simulink model "xy_frequency"  (R2018a)
settings: Solver=VariableStepAuto  StartTime=0.0  StopTime=20  RelTol=1e-3
undefined symbols (not defined in the file): drone, est_c_A, est_c_B, est_c_C, est_c_D, matrix_xA, matrix_xB, matrix_xC, matrix_xD, matrix_yA, matrix_yB, matrix_yC, matrix_yD, regulator_gain_of_attitude, simulation_sampling_ts, vd, vi, vp, xp, yp
libraries: simulink x3
settings Model: Creator=ros  LastModifiedBy=ros

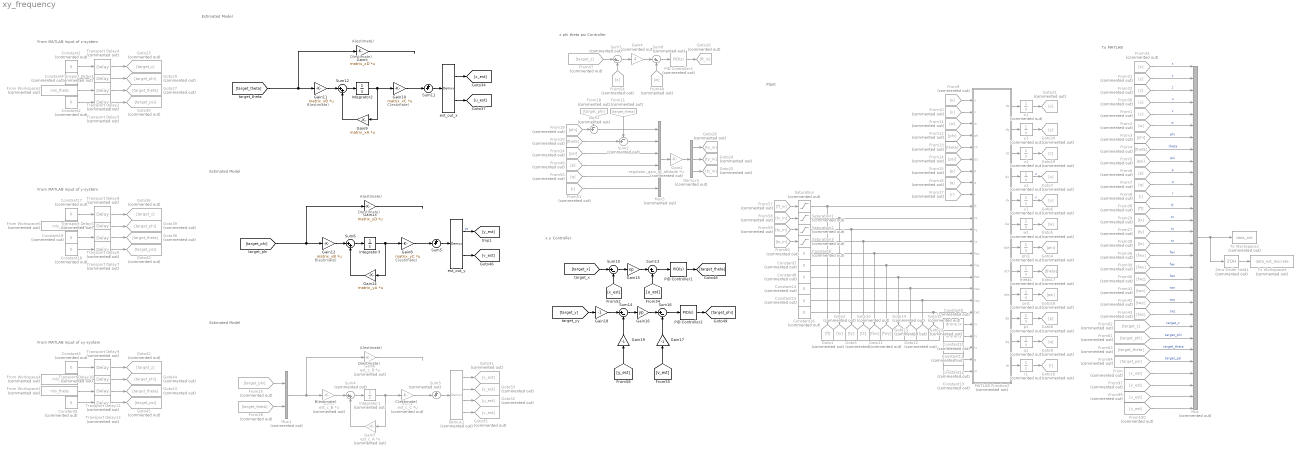
== system xy_frequency ==
  note: To MATLAB
  note: Estimated Model
  note: A(estimate)
  note: B(estimate)
  note: C(estimate)
  note: D(estimate)
  note: z phi theta psi Controller
  note: Plant
  note: D(estimate)
  note: A(estimate)
  note: B(estimate)
  note: Estimated Model
  note: C(estimate)
  note: From MATLAB Input of xy-system
  note: From MATLAB Input of x-system
  note: A(estimate)
  note: B(estimate)
  note: Estimated Model
  note: D(estimate)
  note: C(estimate)
  note: From MATLAB Input of y-system
  note: x y Controller
  Constant{1..8,14..19} (14 alike) : Constant  Commented=on  Value=0
  Constant10 : Constant  Commented=on  Value=drone.Iy
  Constant11 : Constant  Commented=on  Value=drone.Iz
  Constant12 : Constant  Commented=on  Value=drone.g
  Constant13 : Constant  Commented=on  Value=drone.m
  Constant9 : Constant  Commented=on  Value=drone.Ix
  Demux1 : Demux  Commented=on
  Demux5 : Demux  Commented=on  Outputs=3
  From : From  Commented=on  GotoTag=x_est
  From Workspace1 : FromWorkspace  Commented=on  VariableName=mls_theta  SampleTime=0
  From Workspace2 : FromWorkspace  Commented=on  VariableName=mls_theta  SampleTime=0
  From Workspace4 : FromWorkspace  Commented=on  VariableName=mls_phi  SampleTime=0
  From Workspace5 : FromWorkspace  Commented=on  VariableName=mls_phi  SampleTime=0
  From1 : From  Commented=on  GotoTag=v
  From10 : From  Commented=on  GotoTag=v
  From100 : From  Commented=on  GotoTag=v_est
  From11 : From  Commented=on  GotoTag=w
  From12 : From  Commented=on  GotoTag=phi
  From13 : From  Commented=on  GotoTag=theta
  From14 : From  Commented=on  GotoTag=psi
  From15 : From  Commented=on  GotoTag=p
  From16 : From  Commented=on  GotoTag=q
  From17 : From  Commented=on  GotoTag=r
  From18 : From  Commented=on  GotoTag=target_phi
  From19 : From  Commented=on  GotoTag=phi
  From2 : From  Commented=on  GotoTag=w
  From20 : From  Commented=on  GotoTag=theta
  From21 : From  Commented=on  GotoTag=target_theta
  From24 : From  Commented=on  GotoTag=psi
  From25 : From  Commented=on  GotoTag=target_phi
  From26 : From  Commented=on  GotoTag=target_theta
  From27 : From  Commented=on  GotoTag=ty
  From28 : From  Commented=on  GotoTag=tz
  From29 : From  Commented=on  GotoTag=tx
  From3 : From  Commented=on  GotoTag=phi
  From30 : From  Commented=on  GotoTag=u
  From31 : From  Commented=on  GotoTag=y
  From32 : From  Commented=on  GotoTag=z
  From33 : From  Commented=on  GotoTag=x
  From36 : From  Commented=on  GotoTag=fwx
  From38 : From  Commented=on  GotoTag=ft
  From39 : From  Commented=on  GotoTag=fwy
  From4 : From  Commented=on  GotoTag=theta
  From40 : From  Commented=on  GotoTag=fwz
  From41 : From  Commented=on  GotoTag=twx
  From42 : From  Commented=on  GotoTag=twy
  From43 : From  Commented=on  GotoTag=twz
  From47 : From  Commented=on  GotoTag=target_z
  From48 : From  Commented=on  GotoTag=w
  From49 : From  Commented=on  GotoTag=p
  From5 : From  Commented=on  GotoTag=psi
  From50 : From  Commented=on  GotoTag=q
  From51 : From  Commented=on  GotoTag=r
  From54 : From  Commented=on  GotoTag=z
  From57 : From  Commented=on  GotoTag=ft_in
  From58 : From  Commented=on  GotoTag=tx_in
  From59 : From  Commented=on  GotoTag=ty_in
  From6 : From  Commented=on  GotoTag=p
  From60 : From  Commented=on  GotoTag=tz_in
  From61 : From  Commented=on  GotoTag=target_phi
  From62 : From  Commented=on  GotoTag=target_z
  From63 : From  Commented=on  GotoTag=target_theta
  From64 : From  Commented=on  GotoTag=target_psi
  From7 : From  Commented=on  GotoTag=q
  From8 : From  Commented=on  GotoTag=r
  From9 : From  Commented=on  GotoTag=u
  From97 : From  Commented=on  GotoTag=y_est
  From99 : From  Commented=on  GotoTag=u_est
  Gain1 : Gain  Commented=on  Gain=-regulator_gain_of_attitude  Multiplication=Matrix(K*u)
  Gain10 : Gain  Gain=matrix_xC  Multiplication=Matrix(K*u)
  Gain11 : Gain  Gain=matrix_xB  Multiplication=Matrix(K*u)
  Gain12 : Gain  Gain=matrix_yB  Multiplication=Matrix(K*u)
  Gain13 : Gain  Gain=matrix_yD  Multiplication=Matrix(K*u)
  Gain14 : Gain  Gain=matrix_yA  Multiplication=Matrix(K*u)
  Gain15 : Gain  Gain=xp
  Gain16 : Gain  Gain=yp
  Gain17 : Gain  Gain=-1
  Gain18 : Gain  Gain=-1
  Gain19 : Gain  Gain=-1
  Gain2 : Gain  Commented=on  Gain=est_c_C  Multiplication=Matrix(K*u)
  Gain3 : Gain  Commented=on  Gain=est_c_B  Multiplication=Matrix(K*u)
  Gain4 : Gain  Commented=on  Gain=4
  Gain5 : Gain  Gain=matrix_xD  Multiplication=Matrix(K*u)
  Gain6 : Gain  Commented=on  Gain=est_c_D  Multiplication=Matrix(K*u)
  Gain7 : Gain  Commented=on  Gain=est_c_A  Multiplication=Matrix(K*u)
  Gain8 : Gain  Gain=matrix_yC  Multiplication=Matrix(K*u)
  Gain9 : Gain  Gain=matrix_xA  Multiplication=Matrix(K*u)
  Goto1 : Goto  Commented=on  GotoTag=ft
  Goto10 : Goto  Commented=on  GotoTag=tz
  Goto11 : Goto  Commented=on  GotoTag=fwx
  Goto12 : Goto  Commented=on  GotoTag=twx
  Goto13 : Goto  Commented=on  GotoTag=fwy
  Goto14 : Goto  Commented=on  GotoTag=fwz
  Goto15 : Goto  Commented=on  GotoTag=twz
  Goto16 : Goto  Commented=on  GotoTag=r
  Goto17 : Goto  Commented=on  GotoTag=theta
  Goto18 : Goto  Commented=on  GotoTag=psi
  Goto19 : Goto  Commented=on  GotoTag=z
  Goto2 : Goto  Commented=on  GotoTag=tx
  Goto20 : Goto  Commented=on  GotoTag=y
  Goto21 : Goto  Commented=on  GotoTag=x
  Goto22 : Goto  Commented=on  GotoTag=twy
  Goto23 : Goto  Commented=on  GotoTag=target_z
  Goto24 : Goto  Commented=on  GotoTag=ty_in
  Goto25 : Goto  Commented=on  GotoTag=tz_in
  Goto26 : Goto  Commented=on  GotoTag=ft_in
  Goto27 : Goto  Commented=on  GotoTag=target_theta
  Goto28 : Goto  Commented=on  GotoTag=tx_in
  Goto29 : Goto  Commented=on  GotoTag=target_phi
  Goto3 : Goto  Commented=on  GotoTag=ty
  Goto30 : Goto  Commented=on  GotoTag=target_psi
  Goto31 : Goto  Commented=on  GotoTag=x_est
  Goto32 : Goto  Commented=on  GotoTag=u_est
  Goto33 : Goto  Commented=on  GotoTag=y_est
  Goto35 : Goto  Commented=on  GotoTag=v_est
  Goto36 : Goto  Commented=on  GotoTag=target_z
  Goto38 : Goto  Commented=on  GotoTag=target_theta
  Goto39 : Goto  Commented=on  GotoTag=target_phi
  Goto4 : Goto  Commented=on  GotoTag=phi
  Goto40 : Goto  Commented=on  GotoTag=target_psi
  Goto42 : Goto  Commented=on  GotoTag=target_z
  Goto43 : Goto  Commented=on  GotoTag=target_theta
  Goto44 : Goto  Commented=on  GotoTag=target_phi
  Goto45 : Goto  Commented=on  GotoTag=target_psi
  Goto5 : Goto  Commented=on  GotoTag=w
  Goto6 : Goto  Commented=on  GotoTag=v
  Goto7 : Goto  Commented=on  GotoTag=u
  Goto8 : Goto  Commented=on  GotoTag=p
  Goto9 : Goto  Commented=on  GotoTag=q
  Integrator1 : Integrator  Commented=on
  Integrator2 : Integrator
  Integrator3 : Integrator
  MATLAB Function2 : MATLAB Function  Commented=on  TreatAsAtomicUnit=on
  Mux : Mux  Commented=on  Inputs=30
  Mux1 : Mux  Commented=on  Inputs=2
  Mux5 : Mux  Commented=on  Inputs=6
  PID Controller1 : simulink/Continuous/PID Controller  Controller=PID  TimeDomain=Continuous-time  SampleTime=-1  IntegratorMethod=Forward Euler  FilterMethod=Forward Euler  Form=Parallel  UseFilter=on  ControllerParametersSource=internal  P=vp  I=vi  D=vd  N=100  InitialConditionSource=internal  InitialConditionForIntegrator=0  InitialConditionForFilter=0  ExternalReset=none  LimitOutput=off  UpperSaturationLimit=inf  LowerSaturationLimit=-inf  LinearizeAsGain=on  AntiWindupMode=none  Kb=1  TrackingMode=off  Kt=1  PParamMin=[]  PParamMax=[]  IParamMin=[]  IParamMax=[]  DParamMin=[]  DParamMax=[]  NParamMin=[]  NParamMax=[]  KbParamMin=[]  KbParamMax=[]  KtParamMin=[]  KtParamMax=[]  POutMin=[]  POutMax=[]  IOutMin=[]  IOutMax=[]  DOutMin=[]  DOutMax=[]  NOutMin=[]  NOutMax=[]  KbOutMin=[]  KbOutMax=[]  KtOutMin=[]  KtOutMax=[]  IntegratorOutMin=[]  IntegratorOutMax=[]  FilterOutMin=[]  FilterOutMax=[]  SumOutMin=[]  SumOutMax=[]  SumI1OutMin=[]  SumI1OutMax=[]  SumI2OutMin=[]  SumI2OutMax=[]  SumI3OutMin=[]  SumI3OutMax=[]  SumDOutMin=[]  SumDOutMax=[]  SaturationOutMin=[]  SaturationOutMax=[]  IntegratorContinuousStateAttributes=''  IntegratorStateMustResolveToSignalObject=off  IntegratorRTWStateStorageClass=Auto  FilterContinuousStateAttributes=''  FilterStateMustResolveToSignalObject=off  FilterRTWStateStorageClass=Auto  DifferentiatorICPrevScaledInput=0  DifferentiatorOutMin=[]  DifferentiatorOutMax=[]  FilterDiffOutCoefMin=[]  FilterDiffOutCoefMax=[]  SumDenOutMin=[]  SumDenOutMax=[]  SumNumOutMin=[]  SumNumOutMax=[]  ReciprocalOutMin=[]  ReciprocalOutMax=[]  DivideOutMin=[]  DivideOutMax=[]  TunerSelectOption=Transfer Function Based (PID Tuner App)
  PID Controller2 : simulink/Continuous/PID Controller  Controller=PID  TimeDomain=Continuous-time  SampleTime=-1  IntegratorMethod=Forward Euler  FilterMethod=Forward Euler  Form=Parallel  UseFilter=on  ControllerParametersSource=internal  P=vp  I=vi  D=vd  N=113.724914636651  InitialConditionSource=internal  InitialConditionForIntegrator=0  InitialConditionForFilter=0  ExternalReset=none  LimitOutput=off  UpperSaturationLimit=inf  LowerSaturationLimit=-inf  LinearizeAsGain=on  AntiWindupMode=none  Kb=1  TrackingMode=off  Kt=1  PParamMin=[]  PParamMax=[]  IParamMin=[]  IParamMax=[]  DParamMin=[]  DParamMax=[]  NParamMin=[]  NParamMax=[]  KbParamMin=[]  KbParamMax=[]  KtParamMin=[]  KtParamMax=[]  POutMin=[]  POutMax=[]  IOutMin=[]  IOutMax=[]  DOutMin=[]  DOutMax=[]  NOutMin=[]  NOutMax=[]  KbOutMin=[]  KbOutMax=[]  KtOutMin=[]  KtOutMax=[]  IntegratorOutMin=[]  IntegratorOutMax=[]  FilterOutMin=[]  FilterOutMax=[]  SumOutMin=[]  SumOutMax=[]  SumI1OutMin=[]  SumI1OutMax=[]  SumI2OutMin=[]  SumI2OutMax=[]  SumI3OutMin=[]  SumI3OutMax=[]  SumDOutMin=[]  SumDOutMax=[]  SaturationOutMin=[]  SaturationOutMax=[]  IntegratorContinuousStateAttributes=''  IntegratorStateMustResolveToSignalObject=off  IntegratorRTWStateStorageClass=Auto  FilterContinuousStateAttributes=''  FilterStateMustResolveToSignalObject=off  FilterRTWStateStorageClass=Auto  DifferentiatorICPrevScaledInput=0  DifferentiatorOutMin=[]  DifferentiatorOutMax=[]  FilterDiffOutCoefMin=[]  FilterDiffOutCoefMax=[]  SumDenOutMin=[]  SumDenOutMax=[]  SumNumOutMin=[]  SumNumOutMax=[]  ReciprocalOutMin=[]  ReciprocalOutMax=[]  DivideOutMin=[]  DivideOutMax=[]  TunerSelectOption=Transfer Function Based (PID Tuner App)
  PID Controller3 : simulink/Continuous/PID Controller  Commented=on  Controller=PID  TimeDomain=Continuous-time  SampleTime=-1  IntegratorMethod=Forward Euler  FilterMethod=Forward Euler  Form=Parallel  UseFilter=on  ControllerParametersSource=internal  P=7  I=6  D=0.7  N=100  InitialConditionSource=internal  InitialConditionForIntegrator=0  InitialConditionForFilter=0  ExternalReset=none  LimitOutput=off  UpperSaturationLimit=inf  LowerSaturationLimit=-inf  LinearizeAsGain=on  AntiWindupMode=none  Kb=1  TrackingMode=off  Kt=1  PParamMin=[]  PParamMax=[]  IParamMin=[]  IParamMax=[]  DParamMin=[]  DParamMax=[]  NParamMin=[]  NParamMax=[]  KbParamMin=[]  KbParamMax=[]  KtParamMin=[]  KtParamMax=[]  POutMin=[]  POutMax=[]  IOutMin=[]  IOutMax=[]  DOutMin=[]  DOutMax=[]  NOutMin=[]  NOutMax=[]  KbOutMin=[]  KbOutMax=[]  KtOutMin=[]  KtOutMax=[]  IntegratorOutMin=[]  IntegratorOutMax=[]  FilterOutMin=[]  FilterOutMax=[]  SumOutMin=[]  SumOutMax=[]  SumI1OutMin=[]  SumI1OutMax=[]  SumI2OutMin=[]  SumI2OutMax=[]  SumI3OutMin=[]  SumI3OutMax=[]  SumDOutMin=[]  SumDOutMax=[]  SaturationOutMin=[]  SaturationOutMax=[]  IntegratorContinuousStateAttributes=''  IntegratorStateMustResolveToSignalObject=off  IntegratorRTWStateStorageClass=Auto  FilterContinuousStateAttributes=''  FilterStateMustResolveToSignalObject=off  FilterRTWStateStorageClass=Auto  DifferentiatorICPrevScaledInput=0  DifferentiatorOutMin=[]  DifferentiatorOutMax=[]  FilterDiffOutCoefMin=[]  FilterDiffOutCoefMax=[]  SumDenOutMin=[]  SumDenOutMax=[]  SumNumOutMin=[]  SumNumOutMax=[]  ReciprocalOutMin=[]  ReciprocalOutMax=[]  DivideOutMin=[]  DivideOutMax=[]  TunerSelectOption=Transfer Function Based (PID Tuner App)
  Saturation{,1..3} (4 alike) : Saturate  Commented=on  UpperLimit=30  LowerLimit=-100
  Sum1 : Sum  Commented=on  Inputs=-+|
  Sum{10,13..14,16} (4 alike) : Sum  Inputs=|+-
  Sum11 : Sum  Inputs=++|
  Sum12 : Sum  Inputs=|++
  Sum2 : Sum  Commented=on  Inputs=-+|
  Sum3 : Sum  Commented=on  Inputs=++|
  Sum4 : Sum  Commented=on  Inputs=|++
  Sum5 : Sum  Inputs=++|
  Sum6 : Sum  Inputs=|++
  Sum7 : Sum  Commented=on  Inputs=|+-
  Sum8 : Sum  Commented=on  Inputs=|+-
  To Workspace2 : ToWorkspace  Commented=on  VariableName=data_est  SaveFormat=Timeseries  SampleTime=-1
  To Workspace4 : ToWorkspace  Commented=on  VariableName=data_est_discrete  SaveFormat=Timeseries  SampleTime=-1
  Transport Delay{1..12} (12 alike) : TransportDelay  Commented=on  DelayTime=10
  Zero-Order Hold1 : ZeroOrderHold  Commented=on  SampleTime=simulation_sampling_ts
  est_out_x : Demux  Outputs=2
  est_out_y : Demux  Tag=dfd  Outputs=2
  p1 : Integrator  Commented=on
  phi1 : Integrator  Commented=on
  psi1 : Integrator  Commented=on
  q1 : Integrator  Commented=on
  r1 : Integrator  Commented=on
  theta1 : Integrator  Commented=on
  u1 : Integrator  Commented=on
  v1 : Integrator  Commented=on
  w1 : Integrator  Commented=on
  x1 : Integrator  Commented=on
  y1 : Integrator  Commented=on
  z1 : Integrator  Commented=on
  wires:
  From33/1 -> Mux/1  "x"
  From1/1 -> Mux/5  "v"
  From32/1 -> Mux/3  "z"
  From2/1 -> Mux/6  "w"
  From6/1 -> Mux/10  "p"
  From3/1 -> Mux/7  "phi"
  From4/1 -> Mux/8  "theta"
  From8/1 -> Mux/12  "r"
  From31/1 -> Mux/2  "y"
  From5/1 -> Mux/9  "psi"
  From30/1 -> Mux/4  "u"
  From7/1 -> Mux/11  "q"
  Mux/1 -> Zero-Order Hold1/1, To Workspace2/1
  From38/1 -> Mux/13  "ft"
  From29/1 -> Mux/14  "tx"
  From27/1 -> Mux/15  "ty"
  From28/1 -> Mux/16  "tz"
  From36/1 -> Mux/17  "fwx"
  From39/1 -> Mux/18  "fwy"
  From40/1 -> Mux/19  "fwz"
  From41/1 -> Mux/20  "twx"
  From42/1 -> Mux/21  "twy"
  From43/1 -> Mux/22  "twz"
  Zero-Order Hold1/1 -> To Workspace4/1
  From62/1 -> Mux/23  "target_z"
  From61/1 -> Mux/24  "target_phi"
  From63/1 -> Mux/25  "target_theta"
  From64/1 -> Mux/26  "target_psi"
  From/1 -> Mux/27
  From97/1 -> Mux/28
  est_out_x/1 -> [x_est]
  Sum11/1 -> est_out_x/1
  Integrator2/1 -> Gain10/1, Gain9/1
  Gain5/1 -> ?
  Gain11/1 -> Sum12/1
  Gain9/1 -> Sum12/2
  Gain10/1 -> Sum11/2
  Sum12/1 -> Integrator2/1
  [target_theta] -> Gain5/1, Gain11/1
  est_out_x/2 -> [u_est]
  PID Controller3/1 -> Goto26/1
  From47/1 -> Sum7/1
  Sum1/1 -> Mux5/1
  Sum2/1 -> Mux5/2
  From20/1 -> Sum2/2
  Demux5/3 -> Goto25/1
  Sum8/1 -> PID Controller3/1
  From54/1 -> Sum7/2
  Demux5/2 -> Goto24/1
  From51/1 -> Mux5/6
  From50/1 -> Mux5/5
  Demux5/1 -> Goto28/1
  From19/1 -> Sum1/2
  From21/1 -> Sum2/1
  Gain1/1 -> Demux5/1
  Sum7/1 -> Gain4/1
  From18/1 -> Sum1/1
  From48/1 -> Sum8/2
  Mux5/1 -> Gain1/1
  From24/1 -> Mux5/3
  From49/1 -> Mux5/4
  Gain4/1 -> Sum8/1
  v1/1 -> Goto6/1  "v"
  MATLAB Function2/8(dth) -> theta1/1
  From57/1 -> Saturation/1
  MATLAB Function2/10(dp) -> p1/1
  Constant16/1 -> Goto15/1, MATLAB Function2/19(twz)
  MATLAB Function2/12(dr) -> r1/1
  MATLAB Function2/2(dy) -> y1/1
  Constant8/1 -> Goto14/1, MATLAB Function2/16(fwz)
  w1/1 -> Goto5/1
  MATLAB Function2/4(du) -> u1/1
  phi1/1 -> Goto4/1
  Constant15/1 -> Goto22/1, MATLAB Function2/18(twy)
  From16/1 -> MATLAB Function2/8(q)
  From60/1 -> Saturation3/1
  MATLAB Function2/7(dph) -> phi1/1
  Constant6/1 -> Goto11/1, MATLAB Function2/14(fwx)
  Saturation/1 -> Goto1/1, MATLAB Function2/10(ft)
  Saturation3/1 -> Goto10/1, MATLAB Function2/13(tz)
  From12/1 -> MATLAB Function2/4(ph)
  Constant13/1 -> MATLAB Function2/24(m)
  Constant9/1 -> MATLAB Function2/20(Ix)
  z1/1 -> Goto19/1
  q1/1 -> Goto9/1
  psi1/1 -> Goto18/1
  From17/1 -> MATLAB Function2/9(r)
  From13/1 -> MATLAB Function2/5(th)
  MATLAB Function2/5(dv) -> v1/1
  Constant12/1 -> MATLAB Function2/23(g)
  Saturation2/1 -> Goto3/1, MATLAB Function2/12(ty)
  r1/1 -> Goto16/1
  Constant7/1 -> Goto13/1, MATLAB Function2/15(fwy)
  MATLAB Function2/9(dps) -> psi1/1
  Constant11/1 -> MATLAB Function2/22(Iz)
  From15/1 -> MATLAB Function2/7(p)
  theta1/1 -> Goto17/1
  From14/1 -> MATLAB Function2/6(ps)
  x1/1 -> Goto21/1
  MATLAB Function2/3(dz) -> z1/1
  From59/1 -> Saturation2/1
  Constant10/1 -> MATLAB Function2/21(Iy)
  MATLAB Function2/11(dq) -> q1/1
  y1/1 -> Goto20/1
  From11/1 -> MATLAB Function2/3(w)
  From9/1 -> MATLAB Function2/1(u)
  From10/1 -> MATLAB Function2/2(v)
  MATLAB Function2/6(dw) -> w1/1
  u1/1 -> Goto7/1  "u"
  p1/1 -> Goto8/1
  Saturation1/1 -> Goto2/1, MATLAB Function2/11(tx)
  Constant14/1 -> Goto12/1, MATLAB Function2/17(twx)
  MATLAB Function2/1(dx) -> x1/1
  From58/1 -> Saturation1/1
  From100/1 -> Mux/30
  From99/1 -> Mux/29
  Integrator1/1 -> Gain2/1, Gain7/1
  Gain6/1 -> ?
  Demux1/1 -> Goto31/1
  Demux1/2 -> Goto33/1
  Demux1/3 -> Goto32/1
  From26/1 -> Mux1/2
  Mux1/1 -> Gain6/1, Gain3/1
  Demux1/4 -> Goto35/1
  From25/1 -> Mux1/1
  Gain2/1 -> Sum3/2
  Sum3/1 -> Demux1/1
  Sum4/1 -> Integrator1/1
  Gain3/1 -> Sum4/1
  Gain7/1 -> Sum4/2
  Constant5/1 -> Transport Delay12/1
  Constant1/1 -> Transport Delay4/1
  From Workspace1/1 -> Transport Delay11/1
  Transport Delay2/1 -> Goto27/1
  Transport Delay4/1 -> Goto23/1
  From Workspace2/1 -> Transport Delay2/1
  Transport Delay10/1 -> Goto44/1
  Transport Delay3/1 -> Goto30/1
  Constant4/1 -> Transport Delay1/1
  Transport Delay11/1 -> Goto43/1
  Transport Delay1/1 -> Goto29/1
  Transport Delay9/1 -> Goto42/1
  Constant3/1 -> Transport Delay9/1
  Constant2/1 -> Transport Delay3/1
  From Workspace4/1 -> Transport Delay10/1
  Transport Delay12/1 -> Goto45/1
  Gain13/1 -> ?
  est_out_y/1 -> [y_est]  "yo"
  [target_phi] -> Gain13/1, Gain12/1
  Gain8/1 -> Sum5/2
  Integrator3/1 -> Gain8/1, Gain14/1
  est_out_y/2 -> [v_est]
  Sum5/1 -> est_out_y/1
  Sum6/1 -> Integrator3/1
  Gain12/1 -> Sum6/1
  Gain14/1 -> Sum6/2
  Constant18/1 -> Transport Delay7/1
  Transport Delay7/1 -> Goto40/1
  Constant19/1 -> Transport Delay6/1
  Transport Delay8/1 -> Goto36/1
  Transport Delay5/1 -> Goto39/1
  Transport Delay6/1 -> Goto38/1
  Constant17/1 -> Transport Delay8/1
  From Workspace5/1 -> Transport Delay5/1
  PID Controller1/1 -> [target_theta]
  [y_est] -> Gain19/1
  Gain16/1 -> Sum16/1
  [v_est] -> Gain17/1
  Gain15/1 -> Sum13/1
  Sum16/1 -> PID Controller2/1
  [x_est] -> Sum10/2
  PID Controller2/1 -> [target_phi]
  Sum14/1 -> Gain16/1
  [target_y] -> Gain18/1
  [target_x] -> Sum10/1
  Sum13/1 -> PID Controller1/1
  [u_est] -> Sum13/2
  Sum10/1 -> Gain15/1
  Gain18/1 -> Sum14/1
  Gain19/1 -> Sum14/2
  Gain17/1 -> Sum16/2

== matlab function xy_frequency/MATLAB Function2 ==
  data: u input; v input; dx output; w input; ph input; th input; ps input; p input; q input; r input; ft input; tx input; ty input; tz input; fwx input; fwy input; fwz input; twx input; twy input; twz input; dy output; dz output; du output; dv output; dw output; dph output; dth output; dps output; dp output; dq output; dr output; Ix input; Iy input; Iz input; g input; m input
function [dx, dy, dz, du, dv, dw, dph, dth, dps, dp, dq, dr] = fcn(u, v, w, ph, th, ps, p, q, r, ft, tx, ty, tz, fwx, fwy, fwz, twx, twy, twz, Ix, Iy, Iz, g, m)

dx = w*(sin(ph)*sin(ps) + cos(ph)*cos(ps)*sin(th)) - v*(cos(ph)*sin(ps) - cos(ps)*sin(ph)*sin(th)) + u*(cos(ps)*cos(th));
dy = v*(cos(ph)*cos(ps) + sin(ph)*sin(ps)*sin(th)) - w*(cos(ps)*sin(ph) - cos(ph)*sin(ps)*sin(th)) + u*(cos(th)*sin(ps));
dz = w*(cos(ph)*cos(th)) - u*(sin(th)) + v*(cos(th)*sin(ph));
du = r*v - q*w + g*(sin(th)) + fwx / m;
dv = p*w - r*u - g*(sin(ph)*cos(th)) + fwy / m;
dw = q*u - p*v - g*(cos(th)*cos(ph)) + (fwz + ft) / m;
dph = p + r*(cos(ph)*tan(th)) + q*(sin(ph)*tan(th));
dth = q*(cos(th)) - r*(sin(ph));
dps = r*(cos(ph)/cos(th)) + q*(sin(ph)/cos(th));
dp = r*q*(Iy - Iz)/Ix + (tx + twx)/Ix;
dq = p*r*(Iz - Ix)/Iy + (ty + twy)/Iy;
dr = p*q*(Ix - Iy)/Iz + (tz + twz)/Iz;
